simulink model "IDVDSGRA_StatObs_Close"  (R2017b)
settings: Solver=ode4  StartTime=0.0  StopTime=tsim  FixedStep=baseRate  RelTol=1e-3  EnableMultiTasking=on
values from neighbouring files (symbols this model uses):
  baseRate = 0.05    [Run_Initializer.m]
  dockDist = 0.5    [Run_Initializer.m]
  drop_states_BLACK = [ 1.19; 1.45; -0.06737]    [Run_Initializer.m]
  drop_states_RED = [ 2.114; 1.46; -3.113]    [Run_Initializer.m]
  F_thrusters_BLACK = 0.25.*ones(8,1)    [Run_Initializer.m]
  F_thrusters_RED = 0.25.*ones(8,1)    [Run_Initializer.m]
  final_states_BLACK = [1; 0.5; (0/180*pi)]    [Run_Initializer.m]
  fixed_att = init_states_RED(3)    [Run_Initializer.m]
  guess = [8.968203153403679e+02,-2.543974115068790e+03,0.235869606391541,0.474952865321742,0.474987768379695,0.520000000000000,0.485664087948638,0,0,.1,.1,.1,.1,.1,.1,.1,.1,.1,.1,.1,.1,.1,.1,.1,.1,.1,.2]    [Run_Initializer.m]
  home_states_BLACK = [ xLength/2; yLength/2; 0]    [Run_Initializer.m]
  home_states_RED = [ xLength/2+0.4; yLength/2; pi]    [Run_Initializer.m]
  init_states_BLACK = [0.5; 0.5; (0/180*pi)]    [Run_Initializer.m]
  init_states_RED = [ 3; 2; 0]    [Run_Initializer.m]
  Kd_tb = 0.4    [Run_Initializer.m]
  Kd_tr = 0.4    [Run_Initializer.m]
  Kd_xb = 5    [Run_Initializer.m]
  Kd_xr = 5    [Run_Initializer.m]
  Kd_yb = 5    [Run_Initializer.m]
  Kd_yr = 5    [Run_Initializer.m]
  Kp_tb = 0.1    [Run_Initializer.m]
  Kp_tr = 0.1    [Run_Initializer.m]
  Kp_xb = 2    [Run_Initializer.m]
  Kp_xr = 2    [Run_Initializer.m]
  Kp_yb = 2    [Run_Initializer.m]
  Kp_yr = 2    [Run_Initializer.m]
  max_force = F_thrusters_RED(1)*2 * 0.95    [Run_Initializer.m]
  max_torque = 0.13*4    (= 0.52)    [Run_Initializer.m]
  moving_BLACK = [(final_states_BLACK(1)-init_states_BLACK(1))/Phase3_SubPhase2_Duration,(final_states_BLACK(2)-init_states_BLACK(2))/Phase3_SubPhase2_Duration,0]    [Run_Initializer.m]
  noise_variance_BLACK = 0    [Run_Initializer.m]
  noise_variance_RED = 0    [Run_Initializer.m]
  Phase0_End = Phase0_Duration    (= 10)    [Run_Initializer.m]
  Phase1_End = Phase0_Duration + Phase1_Duration    (= 15)    [Run_Initializer.m]
  Phase2_End = Phase0_Duration + Phase1_Duration +                                   Phase2_Duration    (= 35)    [Run_Initializer.m]
  Phase3_Duration = 85    [Run_Initializer.m]
  Phase3_End = Phase0_Duration + Phase1_Duration +                                   Phase2_Duration + Phase3_Duration    (= 120)    [Run_Initializer.m]
  Phase3_SubPhase1_End = Phase2_End + Phase3_SubPhase1_Duration    (= 40)    [Run_Initializer.m]
  Phase3_SubPhase2_Duration = 70    [Run_Initializer.m]
  Phase3_SubPhase2_End = Phase2_End + Phase3_SubPhase1_Duration +                                   Phase3_SubPhase2_Duration    (= 110)    [Run_Initializer.m]
  Phase3_SubPhase3_End = Phase2_End + Phase3_SubPhase1_Duration +                                   Phase3_SubPhase2_Duration +                                  Phase3_SubPhase3_Duration    (= 120)    [Run_Initializer.m]
  Phase3_SubPhase4_End = Phase2_End + Phase3_SubPhase1_Duration +                                   Phase3_SubPhase2_Duration +                                  Phase3_SubPhase3_Duration +                                  Phase3_SubPhase4_Duration    [Run_Initializer.m]
  Phase4_End = Phase0_Duration + Phase1_Duration +                                   Phase2_Duration + Phase3_Duration +                                   Phase4_Duration    (= 140)    [Run_Initializer.m]
  Phase5_End = Phase0_Duration + Phase1_Duration +                                   Phase2_Duration + Phase3_Duration +                                   Phase4_Duration + Phase5_Duration    (= 145)    [Run_Initializer.m]
  REDInertia = 0.2709    [Run_Initializer.m]
  REDMass = 16.9478    [Run_Initializer.m]
  serverRate = 0.1    [Run_Initializer.m]
  thruster_dist2CG_BLACK = [83.42;-52.58;55.94;-60.05;54.08;-53.92;77.06;-55.94]    [Run_Initializer.m]
  thruster_dist2CG_RED = [49.92;-78.08;70.46;-63.54;81.08;-50.42;57.44;-75.96]    [Run_Initializer.m]
  tolSGRA = [Er; Eg]    [Run_Initializer.m]
  xLength = 3.51155    [Run_Initializer.m]
  yLength = 2.41935    [Run_Initializer.m]
undefined symbols (not defined in the file or in its folder): DiscIntNeverNeededParam, platformSelection, simMode
libraries: MainLibrary x22, GPIOLibrary x20, raspberrypilib x17, embdlinuxlib x6, dspsigops x5, dspswit3 x2, simulink x1
(part 7 of 8)

== matlab function IDVDSGRA_StatObs_Close/Phase #3: Experiment/Change RED Behavior/Sub-Phase #2 /Embedded MATLAB Function4 ==
  data: fixed_att input; F output; dock input; cha input; tar input; r0 input; tol input; r output; s input; F0 input; Tmax input; timein input
function [F,r]=IDVD3SGRA(fixed_att, dock,cha,tar,r0,tol,s,F0,Tmax,timein)

%% Definitions of variables
% g = performance index = the manoeuvre's energy [1x1]
% gg = gradient of g [8x1]
% h = constraints [5x1]
% hg = gradient of constraints [8x5]
% g and h are irt varied parameters, r
% r = [d1, d2, tauf, e_FX, e_FY, e_TZ, u, e_t, a4-a9, b4-b9, c4-c9] =[1x26]

% P = constraint error
% E = restoration tolerance 
% cha = chaser's position and velocity [x,y,theta, vx, vy, theta_dot]
% tar = target's position and velocity [x,y,theta, vx, vy, theta_dot]
% dock = docking variables [mass, Ix, FXmax, FYmax, FZmax, docking distance]


if s==0 && Tmax-timein > 1

    Er=tol(1);Eg=tol(2);
    if Tmax-timein>2
        RemTime=Tmax-timein;
    else
        RemTime=2;
    end
    

    par=[dock;cha;tar;RemTime;fixed_att];% Collect all variables in one vector
    
    % Initial Setup
    h = findh(r0, par); 
    P = h' * h;
    Q = 1;
    r=r0;
    
    % Check if Restoration Needed
    if P > Er
            [r, P, Q] = restoration(r, par, P, Er);
    end
  
    % Sequential Algorithm
    loop = 0;
    r_best = r;
    Q_best = Q;

    while loop < 4
        loop = loop + 1;
        [r,P,Q] = gradient(r, par, P, Eg, Q);

        if P > Er
            [r, P, Q] = restoration(r, par, P, Er);
        end

        if (Q < Q_best) && (P <= Er)
            Q_best = Q;
            r_best = r;
        end 
    end
       
    [~,~,~,~,~,~,~,~,F] = final(par, r_best);
    %[tau,t,xt,yt,theta,vx,vy,thetadot,u]=mevalf(par,r_best);
else
    F=zeros(3,1);
    F(1)=F0(1);F(2)=F0(2);F(3)=F0(3);r=r0;
end
end
%%%%%%%%%%%%%%%%%%%%%%%%%%%%%%%%%%%%%%%%%%%%%%%%%%%%%%%%%%%%%%%%%%%%%%%%%%%
%%%%%%%%%%%%%%%%%%%%%%%%%%%%%%%%%%%%%%%%%%%%%%%%%%%%%%%%%%%%%%%%%%%%%%%%%%%
function [r, P, Q] = restoration(r, par, P, Er)
%% Restoration Phase
q=0;
while (P>Er) && (q<10)
    q=q+1;          % counter -> don't do more than 10 iterations
    
    hg = findhg(r, par);
    h = findh(r, par);
    alfa = (hg' * hg) \ h;          % Lagrange multiplier except for the scaling factor, k
    s_delta = -hg * alfa;           % displacement

    k = 1;                          % scaling factor
    qa = 1;
    rp = r + k*s_delta;
    h = findh(rp, par);
    Pp = h'*h;

    while (Pp >= P) && (qa <5)      % using bisection method
        qa = qa +1;                 % only do max 4 iterations
        k = k / 2;
        rp = r + k*s_delta;
        h = findh(rp, par);
        Pp = h'*h;
    end
    r=rp;
    P=Pp;
end

gg = findgg(r, par);
hg = findhg(r, par);
lambda = -(hg' * hg) \ (hg' * gg);
G = gg + hg*lambda;
Q = G' * G;
       
end 
function [r,P,Q] = gradient(r, par, P, Eg, Q)
%% Gradient Phase
count = 0; 
while (Q>Eg) && (count <3)
    count = count + 1;          % no more than 3 iterations   
    
    gg = findgg(r, par);
    hg = findhg(r, par);
    lambda = -(hg' * hg) \ (hg' * gg);
    G = gg + (hg * lambda);
    Q = G' * G;
    
    alfa = 0;
    da = 0.02; 
    
    % Need to find when psi = 0 to find the step size alpha(alfa)
    psi1 = (findgg(r-alfa.*G, par) + (findhg(r-alfa.*G, par)*lambda))' * G ;
    psi2 = (findgg(r-(alfa+da)*G, par) + (findhg(r-(alfa+da)*G, par)*lambda))' * G ;
    
    while (sign(psi1)== sign(psi2)) && (alfa<100) 
        da=da+da^1.3;
        alfa=alfa+da;
        psi1=psi2;
        psi2 = (findgg(r-(alfa+da)*G, par) + (findhg(r-(alfa+da)*G, par)*lambda))' * G ;
    end
    
    alfa = (alfa*psi2 -(alfa+da)*psi1)/(psi2-psi1); % Linear interpolation
    if alfa <= 0         % cannot be a negative number; if it is, set to 1
        alfa = 1;
    end
    
    s = r - alfa*G;
    h = findh(s, par);
    P = h'*h;
    
    Ftilde0 = findg(r, par) + lambda' * findh(r, par);
    count2 = 0;
    hp = h;
    while ((findg(s, par)+lambda'*hp) >= Ftilde0 || P > 10) && (count2<5)
        count2 = count2 + 1;
        alfa = alfa/2;
        s = r-alfa*G;
        hp = findh(s, par);
        P = hp'*hp;
    end    
   
    r = s;
    hg = findhg(r, par);
    gg = findgg(r, par);
    lambda = -(hg' * hg) \ (hg' * gg);
    G = gg + (hg * lambda);
    Q = G' * G;
end  
end 
function [TAU,t,xt,yt,theta,vx,vy,om,F] = final(par, r)
% Performs the final calculations to determine the required thruster
% force in each direction

% Separating out the inputs (computational efficiency)
m=par(1);Iz=par(2);FXmax=par(3);FYmax=par(4);FZmax=par(5);dd=par(6); 
cx=par(7);cy=par(8);cz=par(9);cx_2=par(10);cy_2=par(11);cz_2=par(12);
tx=par(13);ty=par(14);tz=par(15);tx_2=par(16);ty_2=par(17);tz_2=par(18);
Tmax=par(19);fixed_att=par(20);

d1 = r(1); d2 = r(2); tauf = r(3); 
x4=r(9); x5=r(10); x6=r(11); x7=r(12); x8=r(13); x9=r(14);
y4=r(15); y5=r(16); y6=r(17); y7=r(18); y8=r(19); y9=r(20);
z4=r(21); z5=r(22); z6=r(23); z7=r(24); z8=r(25); z9=r(26);

% Initializing 
N=100;
deltaTau = tauf/N;
TAU = zeros(1,N+1);
for i= 2:N+1
    TAU(i) = TAU(i-1) + deltaTau;
end

t=zeros(1,N+1);xt=zeros(1,N+1);yt=zeros(1,N+1);theta=zeros(1,N+1);vx=zeros(1,N+1);
vy=zeros(1,N+1);om=zeros(1,N+1);Fix=zeros(1,N+1);Fiy=zeros(1,N+1);Tz=zeros(1,N+1);

% These equations are the exact same as Marco's (comparison sake), will
% update later
for i = 1:N+1
    tau=TAU(i);
    t(i)=d1*tau+d2*tau^2;
%     xt(i)=cx+cx_2*d1*tau+1/2*(-4*cx_2*d1*tauf-6*cx+6*tx+6*tx_2*(d1*tauf+d2*tauf^2)+6*dd*cos(tz+tz_2*(d1*tauf+d2*tauf^2))-2*tauf*(tx_2-tz_2*dd*sin(tz+tz_2*(d1*tauf+d2*tauf^2)))*(d1+2*d2*tauf))/tauf^2*tau^2+1/6*(12*cx+6*cx_2*d1*tauf-12*tx-12*tx_2*(d1*tauf+d2*tauf^2)-12*dd*cos(tz+tz_2*(d1*tauf+d2*tauf^2))+6*tauf*(tx_2-tz_2*dd*sin(tz+tz_2*(d1*tauf+d2*tauf^2)))*(d1+2*d2*tauf))/tauf^3*tau^3;
%     yt(i)=cy+cy_2*d1*tau+1/2*(-4*cy_2*d1*tauf-6*cy+6*ty+6*ty_2*(d1*tauf+d2*tauf^2)+6*dd*sin(tz+tz_2*(d1*tauf+d2*tauf^2))-2*tauf*(ty_2+tz_2*dd*cos(tz+tz_2*(d1*tauf+d2*tauf^2)))*(d1+2*d2*tauf))/tauf^2*tau^2+1/6*(12*cy+6*cy_2*d1*tauf-12*ty-12*ty_2*(d1*tauf+d2*tauf^2)-12*dd*sin(tz+tz_2*(d1*tauf+d2*tauf^2))+6*tauf*(ty_2+tz_2*dd*cos(tz+tz_2*(d1*tauf+d2*tauf^2)))*(d1+2*d2*tauf))/tauf^3*tau^3;
%     theta(i)=cz+cz_2*d1*tau+1/2*(-4*cz_2*d1*tauf-6*cz+6*tz+6*tz_2*(d1*tauf+d2*tauf^2)-2*tauf*tz_2*(d1+2*d2*tauf))/tauf^2*tau^2+1/6*(12*cz+6*cz_2*d1*tauf-12*tz-12*tz_2*(d1*tauf+d2*tauf^2)+6*tauf*tz_2*(d1+2*d2*tauf))/tauf^3*tau^3;
%     vx(i)=(cx_2*d1+(-4*cx_2*d1*tauf-6*cx+6*tx+6*tx_2*(d1*tauf+d2*tauf^2)+6*dd*cos(tz+tz_2*(d1*tauf+d2*tauf^2))-2*tauf*(tx_2-tz_2*dd*sin(tz+tz_2*(d1*tauf+d2*tauf^2)))*(d1+2*d2*tauf))/tauf^2*tau+1/2*(12*cx+6*cx_2*d1*tauf-12*tx-12*tx_2*(d1*tauf+d2*tauf^2)-12*dd*cos(tz+tz_2*(d1*tauf+d2*tauf^2))+6*tauf*(tx_2-tz_2*dd*sin(tz+tz_2*(d1*tauf+d2*tauf^2)))*(d1+2*d2*tauf))/tauf^3*tau^2)/(d1+2*d2*tau);
%     vy(i)=(cy_2*d1+(-4*cy_2*d1*tauf-6*cy+6*ty+6*ty_2*(d1*tauf+d2*tauf^2)+6*dd*sin(tz+tz_2*(d1*tauf+d2*tauf^2))-2*tauf*(ty_2+tz_2*dd*cos(tz+tz_2*(d1*tauf+d2*tauf^2)))*(d1+2*d2*tauf))/tauf^2*tau+1/2*(12*cy+6*cy_2*d1*tauf-12*ty-12*ty_2*(d1*tauf+d2*tauf^2)-12*dd*sin(tz+tz_2*(d1*tauf+d2*tauf^2))+6*tauf*(ty_2+tz_2*dd*cos(tz+tz_2*(d1*tauf+d2*tauf^2)))*(d1+2*d2*tauf))/tauf^3*tau^2)/(d1+2*d2*tau);
%     om(i)=(cz_2*d1+(-4*cz_2*d1*tauf-6*cz+6*tz+6*tz_2*(d1*tauf+d2*tauf^2)-2*tauf*tz_2*(d1+2*d2*tauf))/tauf^2*tau+1/2*(12*cz+6*cz_2*d1*tauf-12*tz-12*tz_2*(d1*tauf+d2*tauf^2)+6*tauf*tz_2*(d1+2*d2*tauf))/tauf^3*tau^2)/(d1+2*d2*tau);
%     Fix(i)=-2*m*(2*cx_2*d1^2*tauf^2-2*tx_2*tauf^2*d1^2-6*tau^2*cx*d2+6*tau^2*tx*d2+3*tauf*cx*d1-3*tauf*tx*d1-6*tau*cx*d1+6*tau*tx*d1-tauf^2*tz_2*dd*sin(tz+tz_2*d1*tauf+tz_2*d2*tauf^2)*d1^2+6*tauf^2*tz_2*dd*sin(tz+tz_2*d1*tauf+tz_2*d2*tauf^2)*d1*d2*tau-3*tau^2*cx_2*d1*tauf*d2+3*tau^2*tx_2*tauf*d1*d2+3*tau*tauf*tz_2*dd*sin(tz+tz_2*d1*tauf+tz_2*d2*tauf^2)*d1^2+3*tau^2*tauf*tz_2*dd*sin(tz+tz_2*d1*tauf+tz_2*d2*tauf^2)*d1*d2+6*tau^2*tz_2*dd*sin(tz+tz_2*d1*tauf+tz_2*d2*tauf^2)*d2^2*tauf^2-2*tz_2*dd*sin(tz+tz_2*d1*tauf+tz_2*d2*tauf^2)*d2*tauf^3*d1-3*tau*cx_2*d1^2*tauf+3*tau*tx_2*tauf*d1^2+6*tau^2*dd*cos(tz+tz_2*d1*tauf+tz_2*d2*tauf^2)*d2-tx_2*tauf^3*d2*d1-3*tauf*dd*cos(tz+tz_2*d1*tauf+tz_2*d2*tauf^2)*d1+6*tau*dd*cos(tz+tz_2*d1*tauf+tz_2*d2*tauf^2)*d1+d2*cx_2*d1*tauf^3)/tauf^3/(d1+2*d2*tau)^3;
%     Fiy(i)=2*m*(-2*cy_2*d1^2*tauf^2+2*ty_2*tauf^2*d1^2+6*tau^2*cy*d2-6*tau^2*ty*d2-3*tauf*cy*d1+3*tauf*ty*d1+6*tau*cy*d1-6*tau*ty*d1+3*tau*cy_2*d1^2*tauf-3*tau*ty_2*tauf*d1^2-6*tau^2*dd*sin(tz+tz_2*d1*tauf+tz_2*d2*tauf^2)*d2+ty_2*tauf^3*d2*d1+3*tauf*dd*sin(tz+tz_2*d1*tauf+tz_2*d2*tauf^2)*d1-6*tau*dd*sin(tz+tz_2*d1*tauf+tz_2*d2*tauf^2)*d1-d2*cy_2*d1*tauf^3-tauf^2*tz_2*dd*cos(tz+tz_2*d1*tauf+tz_2*d2*tauf^2)*d1^2+6*tauf^2*tz_2*dd*cos(tz+tz_2*d1*tauf+tz_2*d2*tauf^2)*d1*d2*tau+3*tau^2*cy_2*d1*tauf*d2-3*tau^2*ty_2*tauf*d1*d2+3*tau*tauf*tz_2*dd*cos(tz+tz_2*d1*tauf+tz_2*d2*tauf^2)*d1^2+3*tau^2*tauf*tz_2*dd*cos(tz+tz_2*d1*tauf+tz_2*d2*tauf^2)*d1*d2+6*tau^2*tz_2*dd*cos(tz+tz_2*d1*tauf+tz_2*d2*tauf^2)*d2^2*tauf^2-2*tz_2*dd*cos(tz+tz_2*d1*tauf+tz_2*d2*tauf^2)*d2*tauf^3*d1)/tauf^3/(d1+2*d2*tau)^3;
%     Tz(i)=-2*Iz*(-3*tau*cz_2*d1^2*tauf+3*tau*tz_2*d1^2*tauf-tz_2*d2*tauf^3*d1+d2*cz_2*d1*tauf^3+3*tau^2*tz_2*d1*tauf*d2-3*tau^2*cz_2*d1*tauf*d2+2*cz_2*d1^2*tauf^2-2*tz_2*d1^2*tauf^2-6*tau^2*cz*d2+6*tau^2*tz*d2+3*tauf*cz*d1-3*tauf*tz*d1-6*tau*cz*d1+6*tau*tz*d1)/tauf^3/(d1+2*d2*tau)^3;
     % theta(i)= cz + ((d2*tau^2 + d1*tau)^3*(2*cz - 2*tz + 2*tauf^4*z4 + 2*tauf^5*z5 + 2*tauf^6*z6 + 2*tauf^7*z7 + 2*tauf^8*z8 + 2*tauf^9*z9 + cz_2*d1*tauf - d1*tauf*tz_2))/tauf^3 - ((d2*tau^2 + d1*tau)^2*(3*cz - 3*tz + 3*tauf^4*z4 + 3*tauf^5*z5 + 3*tauf^6*z6 + 3*tauf^7*z7 + 3*tauf^8*z8 + 3*tauf^9*z9 - d2*tauf^2*tz_2 + 2*cz_2*d1*tauf - 2*d1*tauf*tz_2))/tauf^2 + cz_2*d1*(d2*tau^2 + d1*tau);
     % Fix(i)= -m*(((30*cx - 30*tx + 30*tauf^4*x4 + 30*tauf^5*x5 + 30*tauf^6*x6 + 30*tauf^7*x7 + 30*tauf^8*x8 + 30*tauf^9*x9 - 30*dd*cos(tz + tz_2*(d2*tauf^2 + d1*tauf)) + 11*d2*tauf^2*tx_2 + 20*cx_2*d1*tauf + d1*tauf*tx_2 - 10*d1*dd*tauf*tz_2*sin(tz + tz_2*(d2*tauf^2 + d1*tauf)) - 20*d2*dd*tauf^2*tz_2*sin(tz + tz_2*(d2*tauf^2 + d1*tauf)))/(5*tauf^2) - (6*tau*(10*cx - 10*tx + 10*tauf^4*x4 + 10*tauf^5*x5 + 10*tauf^6*x6 + 10*tauf^7*x7 + 10*tauf^8*x8 + 10*tauf^9*x9 - 10*dd*cos(tz + tz_2*(d2*tauf^2 + d1*tauf)) + 7*d2*tauf^2*tx_2 + 5*cx_2*d1*tauf + 2*d1*tauf*tx_2 - 5*d1*dd*tauf*tz_2*sin(tz + tz_2*(d2*tauf^2 + d1*tauf)) - 10*d2*dd*tauf^2*tz_2*sin(tz + tz_2*(d2*tauf^2 + d1*tauf))))/(5*tauf^3))/(d1 + 2*d2*tau)^2 + (2*d2*(cx_2*d1 - (tau*(30*cx - 30*tx + 30*tauf^4*x4 + 30*tauf^5*x5 + 30*tauf^6*x6 + 30*tauf^7*x7 + 30*tauf^8*x8 + 30*tauf^9*x9 - 30*dd*cos(tz + tz_2*(d2*tauf^2 + d1*tauf)) + 11*d2*tauf^2*tx_2 + 20*cx_2*d1*tauf + d1*tauf*tx_2 - 10*d1*dd*tauf*tz_2*sin(tz + tz_2*(d2*tauf^2 + d1*tauf)) - 20*d2*dd*tauf^2*tz_2*sin(tz + tz_2*(d2*tauf^2 + d1*tauf))))/(5*tauf^2) + (3*tau^2*(10*cx - 10*tx + 10*tauf^4*x4 + 10*tauf^5*x5 + 10*tauf^6*x6 + 10*tauf^7*x7 + 10*tauf^8*x8 + 10*tauf^9*x9 - 10*dd*cos(tz + tz_2*(d2*tauf^2 + d1*tauf)) + 7*d2*tauf^2*tx_2 + 5*cx_2*d1*tauf + 2*d1*tauf*tx_2 - 5*d1*dd*tauf*tz_2*sin(tz + tz_2*(d2*tauf^2 + d1*tauf)) - 10*d2*dd*tauf^2*tz_2*sin(tz + tz_2*(d2*tauf^2 + d1*tauf))))/(5*tauf^3)))/(d1 + 2*d2*tau)^3);
     % Fiy(i)= -m*(((30*cy - 30*ty - 30*dd*sin(tz + tz_2*(d2*tauf^2 + d1*tauf)) + 30*tauf^4*y4 + 30*tauf^5*y5 + 30*tauf^6*y6 + 30*tauf^7*y7 + 30*tauf^8*y8 + 30*tauf^9*y9 + 11*d2*tauf^2*ty_2 + 20*cy_2*d1*tauf + d1*tauf*ty_2 + 10*d1*dd*tauf*tz_2*sin(tz + tz_2*(d2*tauf^2 + d1*tauf)) + 20*d2*dd*tauf^2*tz_2*sin(tz + tz_2*(d2*tauf^2 + d1*tauf)))/(5*tauf^2) - (6*tau*(10*cy - 10*ty - 10*dd*sin(tz + tz_2*(d2*tauf^2 + d1*tauf)) + 10*tauf^4*y4 + 10*tauf^5*y5 + 10*tauf^6*y6 + 10*tauf^7*y7 + 10*tauf^8*y8 + 10*tauf^9*y9 + 7*d2*tauf^2*ty_2 + 5*cy_2*d1*tauf + 2*d1*tauf*ty_2 + 5*d1*dd*tauf*tz_2*sin(tz + tz_2*(d2*tauf^2 + d1*tauf)) + 10*d2*dd*tauf^2*tz_2*sin(tz + tz_2*(d2*tauf^2 + d1*tauf))))/(5*tauf^3))/(d1 + 2*d2*tau)^2 + (2*d2*(cy_2*d1 - (tau*(30*cy - 30*ty - 30*dd*sin(tz + tz_2*(d2*tauf^2 + d1*tauf)) + 30*tauf^4*y4 + 30*tauf^5*y5 + 30*tauf^6*y6 + 30*tauf^7*y7 + 30*tauf^8*y8 + 30*tauf^9*y9 + 11*d2*tauf^2*ty_2 + 20*cy_2*d1*tauf + d1*tauf*ty_2 + 10*d1*dd*tauf*tz_2*sin(tz + tz_2*(d2*tauf^2 + d1*tauf)) + 20*d2*dd*tauf^2*tz_2*sin(tz + tz_2*(d2*tauf^2 + d1*tauf))))/(5*tauf^2) + (3*tau^2*(10*cy - 10*ty - 10*dd*sin(tz + tz_2*(d2*tauf^2 + d1*tauf)) + 10*tauf^4*y4 + 10*tauf^5*y5 + 10*tauf^6*y6 + 10*tauf^7*y7 + 10*tauf^8*y8 + 10*tauf^9*y9 + 7*d2*tauf^2*ty_2 + 5*cy_2*d1*tauf + 2*d1*tauf*ty_2 + 5*d1*dd*tauf*tz_2*sin(tz + tz_2*(d2*tauf^2 + d1*tauf)) + 10*d2*dd*tauf^2*tz_2*sin(tz + tz_2*(d2*tauf^2 + d1*tauf))))/(5*tauf^3)))/(d1 + 2*d2*tau)^3);
     % Tz(i)= -Iz*(((2*(3*cz - 3*tz + 3*tauf^4*z4 + 3*tauf^5*z5 + 3*tauf^6*z6 + 3*tauf^7*z7 + 3*tauf^8*z8 + 3*tauf^9*z9 - d2*tauf^2*tz_2 + 2*cz_2*d1*tauf - 2*d1*tauf*tz_2))/tauf^2 - (6*tau*(2*cz - 2*tz + 2*tauf^4*z4 + 2*tauf^5*z5 + 2*tauf^6*z6 + 2*tauf^7*z7 + 2*tauf^8*z8 + 2*tauf^9*z9 + cz_2*d1*tauf - d1*tauf*tz_2))/tauf^3)/(d1 + 2*d2*tau)^2 + (2*d2*(cz_2*d1 - (2*tau*(3*cz - 3*tz + 3*tauf^4*z4 + 3*tauf^5*z5 + 3*tauf^6*z6 + 3*tauf^7*z7 + 3*tauf^8*z8 + 3*tauf^9*z9 - d2*tauf^2*tz_2 + 2*cz_2*d1*tauf - 2*d1*tauf*tz_2))/tauf^2 + (3*tau^2*(2*cz - 2*tz + 2*tauf^4*z4 + 2*tauf^5*z5 + 2*tauf^6*z6 + 2*tauf^7*z7 + 2*tauf^8*z8 + 2*tauf^9*z9 + cz_2*d1*tauf - d1*tauf*tz_2))/tauf^3))/(d1 + 2*d2*tau)^3);
theta(i)= cz + ((d2*tau^2 + d1*tau)^3*(2*cz - 2*tz + 2*tauf^4*z4 + 2*tauf^5*z5 + 2*tauf^6*z6 + 2*tauf^7*z7 + 2*tauf^8*z8 + 2*tauf^9*z9 + cz_2*d1*tauf - d1*tauf*tz_2))/tauf^3 - ((d2*tau^2 + d1*tau)^2*(3*cz - 3*tz + 3*tauf^4*z4 + 3*tauf^5*z5 + 3*tauf^6*z6 + 3*tauf^7*z7 + 3*tauf^8*z8 + 3*tauf^9*z9 - d2*tauf^2*tz_2 + 2*cz_2*d1*tauf - 2*d1*tauf*tz_2))/tauf^2 + cz_2*d1*(d2*tau^2 + d1*tau);
      Fix(i)= -m*(((2*(3*cx - 3*tx + 3*tauf^4*x4 + 3*tauf^5*x5 + 3*tauf^6*x6 + 3*tauf^7*x7 + 3*tauf^8*x8 + 3*tauf^9*x9 - 3*dd*cos(tz + tz_2*(d2*tauf^2 + d1*tauf)) - d2*tauf^2*tx_2 + 2*cx_2*d1*tauf - 2*d1*tauf*tx_2 - d1*dd*tauf*tz_2*sin(tz + tz_2*(d2*tauf^2 + d1*tauf)) - 2*d2*dd*tauf^2*tz_2*sin(tz + tz_2*(d2*tauf^2 + d1*tauf))))/tauf^2 - (6*tau*(2*cx - 2*tx + 2*tauf^4*x4 + 2*tauf^5*x5 + 2*tauf^6*x6 + 2*tauf^7*x7 + 2*tauf^8*x8 + 2*tauf^9*x9 - 2*dd*cos(tz + tz_2*(d2*tauf^2 + d1*tauf)) + cx_2*d1*tauf - d1*tauf*tx_2 - d1*dd*tauf*tz_2*sin(tz + tz_2*(d2*tauf^2 + d1*tauf)) - 2*d2*dd*tauf^2*tz_2*sin(tz + tz_2*(d2*tauf^2 + d1*tauf))))/tauf^3)/(d1 + 2*d2*tau)^2 + (2*d2*(cx_2*d1 - (2*tau*(3*cx - 3*tx + 3*tauf^4*x4 + 3*tauf^5*x5 + 3*tauf^6*x6 + 3*tauf^7*x7 + 3*tauf^8*x8 + 3*tauf^9*x9 - 3*dd*cos(tz + tz_2*(d2*tauf^2 + d1*tauf)) - d2*tauf^2*tx_2 + 2*cx_2*d1*tauf - 2*d1*tauf*tx_2 - d1*dd*tauf*tz_2*sin(tz + tz_2*(d2*tauf^2 + d1*tauf)) - 2*d2*dd*tauf^2*tz_2*sin(tz + tz_2*(d2*tauf^2 + d1*tauf))))/tauf^2 + (3*tau^2*(2*cx - 2*tx + 2*tauf^4*x4 + 2*tauf^5*x5 + 2*tauf^6*x6 + 2*tauf^7*x7 + 2*tauf^8*x8 + 2*tauf^9*x9 - 2*dd*cos(tz + tz_2*(d2*tauf^2 + d1*tauf)) + cx_2*d1*tauf - d1*tauf*tx_2 - d1*dd*tauf*tz_2*sin(tz + tz_2*(d2*tauf^2 + d1*tauf)) - 2*d2*dd*tauf^2*tz_2*sin(tz + tz_2*(d2*tauf^2 + d1*tauf))))/tauf^3))/(d1 + 2*d2*tau)^3);
      Fiy(i)= -m*(((2*(3*cy - 3*ty - 3*dd*sin(tz + tz_2*(d2*tauf^2 + d1*tauf)) + 3*tauf^4*y4 + 3*tauf^5*y5 + 3*tauf^6*y6 + 3*tauf^7*y7 + 3*tauf^8*y8 + 3*tauf^9*y9 - d2*tauf^2*ty_2 + 2*cy_2*d1*tauf - 2*d1*tauf*ty_2 + d1*dd*tauf*tz_2*sin(tz + tz_2*(d2*tauf^2 + d1*tauf)) + 2*d2*dd*tauf^2*tz_2*sin(tz + tz_2*(d2*tauf^2 + d1*tauf))))/tauf^2 - (6*tau*(2*cy - 2*ty - 2*dd*sin(tz + tz_2*(d2*tauf^2 + d1*tauf)) + 2*tauf^4*y4 + 2*tauf^5*y5 + 2*tauf^6*y6 + 2*tauf^7*y7 + 2*tauf^8*y8 + 2*tauf^9*y9 + cy_2*d1*tauf - d1*tauf*ty_2 + d1*dd*tauf*tz_2*sin(tz + tz_2*(d2*tauf^2 + d1*tauf)) + 2*d2*dd*tauf^2*tz_2*sin(tz + tz_2*(d2*tauf^2 + d1*tauf))))/tauf^3)/(d1 + 2*d2*tau)^2 + (2*d2*(cy_2*d1 - (2*tau*(3*cy - 3*ty - 3*dd*sin(tz + tz_2*(d2*tauf^2 + d1*tauf)) + 3*tauf^4*y4 + 3*tauf^5*y5 + 3*tauf^6*y6 + 3*tauf^7*y7 + 3*tauf^8*y8 + 3*tauf^9*y9 - d2*tauf^2*ty_2 + 2*cy_2*d1*tauf - 2*d1*tauf*ty_2 + d1*dd*tauf*tz_2*sin(tz + tz_2*(d2*tauf^2 + d1*tauf)) + 2*d2*dd*tauf^2*tz_2*sin(tz + tz_2*(d2*tauf^2 + d1*tauf))))/tauf^2 + (3*tau^2*(2*cy - 2*ty - 2*dd*sin(tz + tz_2*(d2*tauf^2 + d1*tauf)) + 2*tauf^4*y4 + 2*tauf^5*y5 + 2*tauf^6*y6 + 2*tauf^7*y7 + 2*tauf^8*y8 + 2*tauf^9*y9 + cy_2*d1*tauf - d1*tauf*ty_2 + d1*dd*tauf*tz_2*sin(tz + tz_2*(d2*tauf^2 + d1*tauf)) + 2*d2*dd*tauf^2*tz_2*sin(tz + tz_2*(d2*tauf^2 + d1*tauf))))/tauf^3))/(d1 + 2*d2*tau)^3);
      Tz(i)= -Iz*(((2*(3*cz - 3*tz + 3*tauf^4*z4 + 3*tauf^5*z5 + 3*tauf^6*z6 + 3*tauf^7*z7 + 3*tauf^8*z8 + 3*tauf^9*z9 - d2*tauf^2*tz_2 + 2*cz_2*d1*tauf - 2*d1*tauf*tz_2))/tauf^2 - (6*tau*(2*cz - 2*tz + 2*tauf^4*z4 + 2*tauf^5*z5 + 2*tauf^6*z6 + 2*tauf^7*z7 + 2*tauf^8*z8 + 2*tauf^9*z9 + cz_2*d1*tauf - d1*tauf*tz_2))/tauf^3)/(d1 + 2*d2*tau)^2 + (2*d2*(cz_2*d1 - (2*tau*(3*cz - 3*tz + 3*tauf^4*z4 + 3*tauf^5*z5 + 3*tauf^6*z6 + 3*tauf^7*z7 + 3*tauf^8*z8 + 3*tauf^9*z9 - d2*tauf^2*tz_2 + 2*cz_2*d1*tauf - 2*d1*tauf*tz_2))/tauf^2 + (3*tau^2*(2*cz - 2*tz + 2*tauf^4*z4 + 2*tauf^5*z5 + 2*tauf^6*z6 + 2*tauf^7*z7 + 2*tauf^8*z8 + 2*tauf^9*z9 + cz_2*d1*tauf - d1*tauf*tz_2))/tauf^3))/(d1 + 2*d2*tau)^3);
    
end

Fx = Fix.*cos(theta) + Fiy.*sin(theta);
Fy = -Fix.*sin(theta) + Fiy.*cos(theta);

if Fx(1)>FXmax
    Fx(1)=FXmax;
elseif  Fx(1)<-FXmax
    Fx(1)=-FXmax;
end

if Fy(1)>FYmax
    Fy(1)=FYmax;
elseif  Fy(1)<-FYmax
    Fy(1)=-FYmax;
end

if Tz(1)>FZmax
    Tz(1)=FZmax;
elseif  Tz(1)<-FZmax
    Tz(1)=-FZmax;
end

F=[Fx(1) Fy(1) Tz(1)]';

end
%%%%%%%%%%%%%%%%%%%%%%%%%%%%%%%%%%%%%%%%%%%%%%%%%%%%%%%%%%%%%%%%%%%%%%%%%%%
function g = findg(r, par)
% This function calculates the performance index 
%
% Inputs:
%   - r = varied parameters = [d1, d2, tauf, e_FX, e_FY, e_TZ, u, e_t]
%   - cha = conditions of chaser 'initial' [x,y,z,xv,yv,zv]
%   - tar = conditions of target 'final' [X,Y,Z,XV,YV,ZV]
%   - dock = docking variables [mass, mom_inertia, Fmax, Torque_max, dock_distance,
%            time_remaining]
% Outputs:
%   - g = performace index [1x1]
% Comment: 

% Separating out the inputs (computational efficiency)
m=par(1);Iz=par(2);FXmax=par(3);FYmax=par(4);FZmax=par(5);dd=par(6); 
cx=par(7);cy=par(8);cz=par(9);cx_2=par(10);cy_2=par(11);cz_2=par(12);
tx=par(13);ty=par(14);tz=par(15);tx_2=par(16);ty_2=par(17);tz_2=par(18);
Tmax=par(19);fixed_att=par(20);

d1 = r(1); d2 = r(2); tauf = r(3); e_FX = r(4);
e_FY = r(5); e_TZ = r(6); u = r(7); e_t = r(8);
x4=r(9); x5=r(10); x6=r(11); x7=r(12); x8=r(13); x9=r(14);
y4=r(15); y5=r(16); y6=r(17); y7=r(18); y8=r(19); y9=r(20);
z4=r(21); z5=r(22); z6=r(23); z7=r(24); z8=r(25); z9=r(26);


% Determining the performance index
n=20;
TAU=(0:1/n:1)*tauf;
fx=zeros(1,length(TAU)); fy=zeros(1,length(TAU)); fz=zeros(1,length(TAU)); E=zeros(1,length(TAU));
    
for i=1:length(TAU)
    tau=TAU(i);
    fx(i)= -m*(((30*cx - 30*tx + 30*tauf^4*x4 + 30*tauf^5*x5 + 30*tauf^6*x6 + 30*tauf^7*x7 + 30*tauf^8*x8 + 30*tauf^9*x9 - 30*dd*cos(tz + tz_2*(d2*tauf^2 + d1*tauf)) + 11*d2*tauf^2*tx_2 + 20*cx_2*d1*tauf + d1*tauf*tx_2 - 10*d1*dd*tauf*tz_2*sin(tz + tz_2*(d2*tauf^2 + d1*tauf)) - 20*d2*dd*tauf^2*tz_2*sin(tz + tz_2*(d2*tauf^2 + d1*tauf)))/(5*tauf^2) - (6*tau*(10*cx - 10*tx + 10*tauf^4*x4 + 10*tauf^5*x5 + 10*tauf^6*x6 + 10*tauf^7*x7 + 10*tauf^8*x8 + 10*tauf^9*x9 - 10*dd*cos(tz + tz_2*(d2*tauf^2 + d1*tauf)) + 7*d2*tauf^2*tx_2 + 5*cx_2*d1*tauf + 2*d1*tauf*tx_2 - 5*d1*dd*tauf*tz_2*sin(tz + tz_2*(d2*tauf^2 + d1*tauf)) - 10*d2*dd*tauf^2*tz_2*sin(tz + tz_2*(d2*tauf^2 + d1*tauf))))/(5*tauf^3))/(d1 + 2*d2*tau)^2 + (2*d2*(cx_2*d1 - (tau*(30*cx - 30*tx + 30*tauf^4*x4 + 30*tauf^5*x5 + 30*tauf^6*x6 + 30*tauf^7*x7 + 30*tauf^8*x8 + 30*tauf^9*x9 - 30*dd*cos(tz + tz_2*(d2*tauf^2 + d1*tauf)) + 11*d2*tauf^2*tx_2 + 20*cx_2*d1*tauf + d1*tauf*tx_2 - 10*d1*dd*tauf*tz_2*sin(tz + tz_2*(d2*tauf^2 + d1*tauf)) - 20*d2*dd*tauf^2*tz_2*sin(tz + tz_2*(d2*tauf^2 + d1*tauf))))/(5*tauf^2) + (3*tau^2*(10*cx - 10*tx + 10*tauf^4*x4 + 10*tauf^5*x5 + 10*tauf^6*x6 + 10*tauf^7*x7 + 10*tauf^8*x8 + 10*tauf^9*x9 - 10*dd*cos(tz + tz_2*(d2*tauf^2 + d1*tauf)) + 7*d2*tauf^2*tx_2 + 5*cx_2*d1*tauf + 2*d1*tauf*tx_2 - 5*d1*dd*tauf*tz_2*sin(tz + tz_2*(d2*tauf^2 + d1*tauf)) - 10*d2*dd*tauf^2*tz_2*sin(tz + tz_2*(d2*tauf^2 + d1*tauf))))/(5*tauf^3)))/(d1 + 2*d2*tau)^3);
    fy(i)= -m*(((30*cy - 30*ty - 30*dd*sin(tz + tz_2*(d2*tauf^2 + d1*tauf)) + 30*tauf^4*y4 + 30*tauf^5*y5 + 30*tauf^6*y6 + 30*tauf^7*y7 + 30*tauf^8*y8 + 30*tauf^9*y9 + 11*d2*tauf^2*ty_2 + 20*cy_2*d1*tauf + d1*tauf*ty_2 + 10*d1*dd*tauf*tz_2*sin(tz + tz_2*(d2*tauf^2 + d1*tauf)) + 20*d2*dd*tauf^2*tz_2*sin(tz + tz_2*(d2*tauf^2 + d1*tauf)))/(5*tauf^2) - (6*tau*(10*cy - 10*ty - 10*dd*sin(tz + tz_2*(d2*tauf^2 + d1*tauf)) + 10*tauf^4*y4 + 10*tauf^5*y5 + 10*tauf^6*y6 + 10*tauf^7*y7 + 10*tauf^8*y8 + 10*tauf^9*y9 + 7*d2*tauf^2*ty_2 + 5*cy_2*d1*tauf + 2*d1*tauf*ty_2 + 5*d1*dd*tauf*tz_2*sin(tz + tz_2*(d2*tauf^2 + d1*tauf)) + 10*d2*dd*tauf^2*tz_2*sin(tz + tz_2*(d2*tauf^2 + d1*tauf))))/(5*tauf^3))/(d1 + 2*d2*tau)^2 + (2*d2*(cy_2*d1 - (tau*(30*cy - 30*ty - 30*dd*sin(tz + tz_2*(d2*tauf^2 + d1*tauf)) + 30*tauf^4*y4 + 30*tauf^5*y5 + 30*tauf^6*y6 + 30*tauf^7*y7 + 30*tauf^8*y8 + 30*tauf^9*y9 + 11*d2*tauf^2*ty_2 + 20*cy_2*d1*tauf + d1*tauf*ty_2 + 10*d1*dd*tauf*tz_2*sin(tz + tz_2*(d2*tauf^2 + d1*tauf)) + 20*d2*dd*tauf^2*tz_2*sin(tz + tz_2*(d2*tauf^2 + d1*tauf))))/(5*tauf^2) + (3*tau^2*(10*cy - 10*ty - 10*dd*sin(tz + tz_2*(d2*tauf^2 + d1*tauf)) + 10*tauf^4*y4 + 10*tauf^5*y5 + 10*tauf^6*y6 + 10*tauf^7*y7 + 10*tauf^8*y8 + 10*tauf^9*y9 + 7*d2*tauf^2*ty_2 + 5*cy_2*d1*tauf + 2*d1*tauf*ty_2 + 5*d1*dd*tauf*tz_2*sin(tz + tz_2*(d2*tauf^2 + d1*tauf)) + 10*d2*dd*tauf^2*tz_2*sin(tz + tz_2*(d2*tauf^2 + d1*tauf))))/(5*tauf^3)))/(d1 + 2*d2*tau)^3);
    fz(i)= -Iz*(((2*(3*cz - 3*tz + 3*tauf^4*z4 + 3*tauf^5*z5 + 3*tauf^6*z6 + 3*tauf^7*z7 + 3*tauf^8*z8 + 3*tauf^9*z9 - d2*tauf^2*tz_2 + 2*cz_2*d1*tauf - 2*d1*tauf*tz_2))/tauf^2 - (6*tau*(2*cz - 2*tz + 2*tauf^4*z4 + 2*tauf^5*z5 + 2*tauf^6*z6 + 2*tauf^7*z7 + 2*tauf^8*z8 + 2*tauf^9*z9 + cz_2*d1*tauf - d1*tauf*tz_2))/tauf^3)/(d1 + 2*d2*tau)^2 + (2*d2*(cz_2*d1 - (2*tau*(3*cz - 3*tz + 3*tauf^4*z4 + 3*tauf^5*z5 + 3*tauf^6*z6 + 3*tauf^7*z7 + 3*tauf^8*z8 + 3*tauf^9*z9 - d2*tauf^2*tz_2 + 2*cz_2*d1*tauf - 2*d1*tauf*tz_2))/tauf^2 + (3*tau^2*(2*cz - 2*tz + 2*tauf^4*z4 + 2*tauf^5*z5 + 2*tauf^6*z6 + 2*tauf^7*z7 + 2*tauf^8*z8 + 2*tauf^9*z9 + cz_2*d1*tauf - d1*tauf*tz_2))/tauf^3))/(d1 + 2*d2*tau)^3);
    E(i)=(fx(i)^2+fy(i)^2+fz(i)^2);
end 

g=trapz(TAU,E.*(d1+2*d2*TAU));

end 
function gg = findgg(r,par)

% Separating out the inputs (computational efficiency)
m=par(1);Iz=par(2);FXmax=par(3);FYmax=par(4);FZmax=par(5);dd=par(6); 
cx=par(7);cy=par(8);cz=par(9);cx_2=par(10);cy_2=par(11);cz_2=par(12);
tx=par(13);ty=par(14);tz=par(15);tx_2=par(16);ty_2=par(17);tz_2=par(18);
Tmax=par(19);fixed_att=par(20);

%%
r = r';
r0 = r;
n=20;
D=abs(r/1000)+0.0001;
dg=zeros(1,length(r));
for j=1:length(r)
    rp=r0; rn=r0;
    rp(j)=rp(j)+D(j);rn(j)=rn(j)-D(j);
    rpn=[rp;rn]; 
    Ep=zeros(1,n+1);En=zeros(1,n+1);
    TAU=(0:1/n:1)*r(3);        
    for s=1:2    % run through the loop twice, once for rp and once for rn
        r=rpn(s,:);
        d1 = r(1); d2 = r(2); tauf = r(3); e_FX = r(4);
        e_FY = r(5); e_TZ = r(6); u = r(7); e_t = r(8);
        x4=r(9); x5=r(10); x6=r(11); x7=r(12); x8=r(13); x9=r(14);
        y4=r(15); y5=r(16); y6=r(17); y7=r(18); y8=r(19); y9=r(20);
        z4=r(21); z5=r(22); z6=r(23); z7=r(24); z8=r(25); z9=r(26);
        
        TAU=(0:1/n:1)*tauf;
        fx=zeros(1,length(TAU)); fy=zeros(1,length(TAU)); fz=zeros(1,length(TAU));
        for i=1:length(TAU)
            tau=TAU(i);
            fx(i)= -m*(((30*cx - 30*tx + 30*tauf^4*x4 + 30*tauf^5*x5 + 30*tauf^6*x6 + 30*tauf^7*x7 + 30*tauf^8*x8 + 30*tauf^9*x9 - 30*dd*cos(tz + tz_2*(d2*tauf^2 + d1*tauf)) + 11*d2*tauf^2*tx_2 + 20*cx_2*d1*tauf + d1*tauf*tx_2 - 10*d1*dd*tauf*tz_2*sin(tz + tz_2*(d2*tauf^2 + d1*tauf)) - 20*d2*dd*tauf^2*tz_2*sin(tz + tz_2*(d2*tauf^2 + d1*tauf)))/(5*tauf^2) - (6*tau*(10*cx - 10*tx + 10*tauf^4*x4 + 10*tauf^5*x5 + 10*tauf^6*x6 + 10*tauf^7*x7 + 10*tauf^8*x8 + 10*tauf^9*x9 - 10*dd*cos(tz + tz_2*(d2*tauf^2 + d1*tauf)) + 7*d2*tauf^2*tx_2 + 5*cx_2*d1*tauf + 2*d1*tauf*tx_2 - 5*d1*dd*tauf*tz_2*sin(tz + tz_2*(d2*tauf^2 + d1*tauf)) - 10*d2*dd*tauf^2*tz_2*sin(tz + tz_2*(d2*tauf^2 + d1*tauf))))/(5*tauf^3))/(d1 + 2*d2*tau)^2 + (2*d2*(cx_2*d1 - (tau*(30*cx - 30*tx + 30*tauf^4*x4 + 30*tauf^5*x5 + 30*tauf^6*x6 + 30*tauf^7*x7 + 30*tauf^8*x8 + 30*tauf^9*x9 - 30*dd*cos(tz + tz_2*(d2*tauf^2 + d1*tauf)) + 11*d2*tauf^2*tx_2 + 20*cx_2*d1*tauf + d1*tauf*tx_2 - 10*d1*dd*tauf*tz_2*sin(tz + tz_2*(d2*tauf^2 + d1*tauf)) - 20*d2*dd*tauf^2*tz_2*sin(tz + tz_2*(d2*tauf^2 + d1*tauf))))/(5*tauf^2) + (3*tau^2*(10*cx - 10*tx + 10*tauf^4*x4 + 10*tauf^5*x5 + 10*tauf^6*x6 + 10*tauf^7*x7 + 10*tauf^8*x8 + 10*tauf^9*x9 - 10*dd*cos(tz + tz_2*(d2*tauf^2 + d1*tauf)) + 7*d2*tauf^2*tx_2 + 5*cx_2*d1*tauf + 2*d1*tauf*tx_2 - 5*d1*dd*tauf*tz_2*sin(tz + tz_2*(d2*tauf^2 + d1*tauf)) - 10*d2*dd*tauf^2*tz_2*sin(tz + tz_2*(d2*tauf^2 + d1*tauf))))/(5*tauf^3)))/(d1 + 2*d2*tau)^3);
            fy(i)= -m*(((30*cy - 30*ty - 30*dd*sin(tz + tz_2*(d2*tauf^2 + d1*tauf)) + 30*tauf^4*y4 + 30*tauf^5*y5 + 30*tauf^6*y6 + 30*tauf^7*y7 + 30*tauf^8*y8 + 30*tauf^9*y9 + 11*d2*tauf^2*ty_2 + 20*cy_2*d1*tauf + d1*tauf*ty_2 + 10*d1*dd*tauf*tz_2*sin(tz + tz_2*(d2*tauf^2 + d1*tauf)) + 20*d2*dd*tauf^2*tz_2*sin(tz + tz_2*(d2*tauf^2 + d1*tauf)))/(5*tauf^2) - (6*tau*(10*cy - 10*ty - 10*dd*sin(tz + tz_2*(d2*tauf^2 + d1*tauf)) + 10*tauf^4*y4 + 10*tauf^5*y5 + 10*tauf^6*y6 + 10*tauf^7*y7 + 10*tauf^8*y8 + 10*tauf^9*y9 + 7*d2*tauf^2*ty_2 + 5*cy_2*d1*tauf + 2*d1*tauf*ty_2 + 5*d1*dd*tauf*tz_2*sin(tz + tz_2*(d2*tauf^2 + d1*tauf)) + 10*d2*dd*tauf^2*tz_2*sin(tz + tz_2*(d2*tauf^2 + d1*tauf))))/(5*tauf^3))/(d1 + 2*d2*tau)^2 + (2*d2*(cy_2*d1 - (tau*(30*cy - 30*ty - 30*dd*sin(tz + tz_2*(d2*tauf^2 + d1*tauf)) + 30*tauf^4*y4 + 30*tauf^5*y5 + 30*tauf^6*y6 + 30*tauf^7*y7 + 30*tauf^8*y8 + 30*tauf^9*y9 + 11*d2*tauf^2*ty_2 + 20*cy_2*d1*tauf + d1*tauf*ty_2 + 10*d1*dd*tauf*tz_2*sin(tz + tz_2*(d2*tauf^2 + d1*tauf)) + 20*d2*dd*tauf^2*tz_2*sin(tz + tz_2*(d2*tauf^2 + d1*tauf))))/(5*tauf^2) + (3*tau^2*(10*cy - 10*ty - 10*dd*sin(tz + tz_2*(d2*tauf^2 + d1*tauf)) + 10*tauf^4*y4 + 10*tauf^5*y5 + 10*tauf^6*y6 + 10*tauf^7*y7 + 10*tauf^8*y8 + 10*tauf^9*y9 + 7*d2*tauf^2*ty_2 + 5*cy_2*d1*tauf + 2*d1*tauf*ty_2 + 5*d1*dd*tauf*tz_2*sin(tz + tz_2*(d2*tauf^2 + d1*tauf)) + 10*d2*dd*tauf^2*tz_2*sin(tz + tz_2*(d2*tauf^2 + d1*tauf))))/(5*tauf^3)))/(d1 + 2*d2*tau)^3);
            fz(i)= -Iz*(((2*(3*cz - 3*tz + 3*tauf^4*z4 + 3*tauf^5*z5 + 3*tauf^6*z6 + 3*tauf^7*z7 + 3*tauf^8*z8 + 3*tauf^9*z9 - d2*tauf^2*tz_2 + 2*cz_2*d1*tauf - 2*d1*tauf*tz_2))/tauf^2 - (6*tau*(2*cz - 2*tz + 2*tauf^4*z4 + 2*tauf^5*z5 + 2*tauf^6*z6 + 2*tauf^7*z7 + 2*tauf^8*z8 + 2*tauf^9*z9 + cz_2*d1*tauf - d1*tauf*tz_2))/tauf^3)/(d1 + 2*d2*tau)^2 + (2*d2*(cz_2*d1 - (2*tau*(3*cz - 3*tz + 3*tauf^4*z4 + 3*tauf^5*z5 + 3*tauf^6*z6 + 3*tauf^7*z7 + 3*tauf^8*z8 + 3*tauf^9*z9 - d2*tauf^2*tz_2 + 2*cz_2*d1*tauf - 2*d1*tauf*tz_2))/tauf^2 + (3*tau^2*(2*cz - 2*tz + 2*tauf^4*z4 + 2*tauf^5*z5 + 2*tauf^6*z6 + 2*tauf^7*z7 + 2*tauf^8*z8 + 2*tauf^9*z9 + cz_2*d1*tauf - d1*tauf*tz_2))/tauf^3))/(d1 + 2*d2*tau)^3);

            if s==1    % 1st run, calculate Ep with rp
                Ep(i)=(fx(i)^2+fy(i)^2+fz(i)^2);
            elseif s==2 % 2nd run, calculate En with rn
                En(i)=(fx(i)^2+fy(i)^2+fz(i)^2);
            end
        end 
    end
    gp=trapz(TAU,Ep.*(d1+2*d2*TAU));
    gn=trapz(TAU,En.*(d1+2*d2*TAU));
    dg(1,j)=(gp-gn)/(2*D(j));
end 

gg=dg';


end 
function h = findh(r, par) 

% Separating out the inputs (computational efficiency)
m=par(1);Iz=par(2);FXmax=par(3);FYmax=par(4);FZmax=par(5);dd=par(6); 
cx=par(7);cy=par(8);cz=par(9);cx_2=par(10);cy_2=par(11);cz_2=par(12);
tx=par(13);ty=par(14);tz=par(15);tx_2=par(16);ty_2=par(17);tz_2=par(18);
Tmax=par(19);fixed_att=par(20);

d1 = r(1); d2 = r(2); tauf = r(3); e_FX = r(4);
e_FY = r(5); e_TZ = r(6); u = r(7); e_t = r(8);
x4=r(9); x5=r(10); x6=r(11); x7=r(12); x8=r(13); x9=r(14);
y4=r(15); y5=r(16); y6=r(17); y7=r(18); y8=r(19); y9=r(20);
z4=r(21); z5=r(22); z6=r(23); z7=r(24); z8=r(25); z9=r(26);

%%
n=20;
TAU=[0:1/n:1]*tauf;
fx=zeros(1,length(TAU));fy=zeros(1,length(TAU));fz=zeros(1,length(TAU));
theta=zeros(1,length(TAU));h=zeros(5,1);
for i=1:length(TAU)
    tau=TAU(i);
    fx(i)= -m*(((30*cx - 30*tx + 30*tauf^4*x4 + 30*tauf^5*x5 + 30*tauf^6*x6 + 30*tauf^7*x7 + 30*tauf^8*x8 + 30*tauf^9*x9 - 30*dd*cos(tz + tz_2*(d2*tauf^2 + d1*tauf)) + 11*d2*tauf^2*tx_2 + 20*cx_2*d1*tauf + d1*tauf*tx_2 - 10*d1*dd*tauf*tz_2*sin(tz + tz_2*(d2*tauf^2 + d1*tauf)) - 20*d2*dd*tauf^2*tz_2*sin(tz + tz_2*(d2*tauf^2 + d1*tauf)))/(5*tauf^2) - (6*tau*(10*cx - 10*tx + 10*tauf^4*x4 + 10*tauf^5*x5 + 10*tauf^6*x6 + 10*tauf^7*x7 + 10*tauf^8*x8 + 10*tauf^9*x9 - 10*dd*cos(tz + tz_2*(d2*tauf^2 + d1*tauf)) + 7*d2*tauf^2*tx_2 + 5*cx_2*d1*tauf + 2*d1*tauf*tx_2 - 5*d1*dd*tauf*tz_2*sin(tz + tz_2*(d2*tauf^2 + d1*tauf)) - 10*d2*dd*tauf^2*tz_2*sin(tz + tz_2*(d2*tauf^2 + d1*tauf))))/(5*tauf^3))/(d1 + 2*d2*tau)^2 + (2*d2*(cx_2*d1 - (tau*(30*cx - 30*tx + 30*tauf^4*x4 + 30*tauf^5*x5 + 30*tauf^6*x6 + 30*tauf^7*x7 + 30*tauf^8*x8 + 30*tauf^9*x9 - 30*dd*cos(tz + tz_2*(d2*tauf^2 + d1*tauf)) + 11*d2*tauf^2*tx_2 + 20*cx_2*d1*tauf + d1*tauf*tx_2 - 10*d1*dd*tauf*tz_2*sin(tz + tz_2*(d2*tauf^2 + d1*tauf)) - 20*d2*dd*tauf^2*tz_2*sin(tz + tz_2*(d2*tauf^2 + d1*tauf))))/(5*tauf^2) + (3*tau^2*(10*cx - 10*tx + 10*tauf^4*x4 + 10*tauf^5*x5 + 10*tauf^6*x6 + 10*tauf^7*x7 + 10*tauf^8*x8 + 10*tauf^9*x9 - 10*dd*cos(tz + tz_2*(d2*tauf^2 + d1*tauf)) + 7*d2*tauf^2*tx_2 + 5*cx_2*d1*tauf + 2*d1*tauf*tx_2 - 5*d1*dd*tauf*tz_2*sin(tz + tz_2*(d2*tauf^2 + d1*tauf)) - 10*d2*dd*tauf^2*tz_2*sin(tz + tz_2*(d2*tauf^2 + d1*tauf))))/(5*tauf^3)))/(d1 + 2*d2*tau)^3);
    fy(i)= -m*(((30*cy - 30*ty - 30*dd*sin(tz + tz_2*(d2*tauf^2 + d1*tauf)) + 30*tauf^4*y4 + 30*tauf^5*y5 + 30*tauf^6*y6 + 30*tauf^7*y7 + 30*tauf^8*y8 + 30*tauf^9*y9 + 11*d2*tauf^2*ty_2 + 20*cy_2*d1*tauf + d1*tauf*ty_2 + 10*d1*dd*tauf*tz_2*sin(tz + tz_2*(d2*tauf^2 + d1*tauf)) + 20*d2*dd*tauf^2*tz_2*sin(tz + tz_2*(d2*tauf^2 + d1*tauf)))/(5*tauf^2) - (6*tau*(10*cy - 10*ty - 10*dd*sin(tz + tz_2*(d2*tauf^2 + d1*tauf)) + 10*tauf^4*y4 + 10*tauf^5*y5 + 10*tauf^6*y6 + 10*tauf^7*y7 + 10*tauf^8*y8 + 10*tauf^9*y9 + 7*d2*tauf^2*ty_2 + 5*cy_2*d1*tauf + 2*d1*tauf*ty_2 + 5*d1*dd*tauf*tz_2*sin(tz + tz_2*(d2*tauf^2 + d1*tauf)) + 10*d2*dd*tauf^2*tz_2*sin(tz + tz_2*(d2*tauf^2 + d1*tauf))))/(5*tauf^3))/(d1 + 2*d2*tau)^2 + (2*d2*(cy_2*d1 - (tau*(30*cy - 30*ty - 30*dd*sin(tz + tz_2*(d2*tauf^2 + d1*tauf)) + 30*tauf^4*y4 + 30*tauf^5*y5 + 30*tauf^6*y6 + 30*tauf^7*y7 + 30*tauf^8*y8 + 30*tauf^9*y9 + 11*d2*tauf^2*ty_2 + 20*cy_2*d1*tauf + d1*tauf*ty_2 + 10*d1*dd*tauf*tz_2*sin(tz + tz_2*(d2*tauf^2 + d1*tauf)) + 20*d2*dd*tauf^2*tz_2*sin(tz + tz_2*(d2*tauf^2 + d1*tauf))))/(5*tauf^2) + (3*tau^2*(10*cy - 10*ty - 10*dd*sin(tz + tz_2*(d2*tauf^2 + d1*tauf)) + 10*tauf^4*y4 + 10*tauf^5*y5 + 10*tauf^6*y6 + 10*tauf^7*y7 + 10*tauf^8*y8 + 10*tauf^9*y9 + 7*d2*tauf^2*ty_2 + 5*cy_2*d1*tauf + 2*d1*tauf*ty_2 + 5*d1*dd*tauf*tz_2*sin(tz + tz_2*(d2*tauf^2 + d1*tauf)) + 10*d2*dd*tauf^2*tz_2*sin(tz + tz_2*(d2*tauf^2 + d1*tauf))))/(5*tauf^3)))/(d1 + 2*d2*tau)^3);
    fz(i)= -Iz*(((2*(3*cz - 3*tz + 3*tauf^4*z4 + 3*tauf^5*z5 + 3*tauf^6*z6 + 3*tauf^7*z7 + 3*tauf^8*z8 + 3*tauf^9*z9 - d2*tauf^2*tz_2 + 2*cz_2*d1*tauf - 2*d1*tauf*tz_2))/tauf^2 - (6*tau*(2*cz - 2*tz + 2*tauf^4*z4 + 2*tauf^5*z5 + 2*tauf^6*z6 + 2*tauf^7*z7 + 2*tauf^8*z8 + 2*tauf^9*z9 + cz_2*d1*tauf - d1*tauf*tz_2))/tauf^3)/(d1 + 2*d2*tau)^2 + (2*d2*(cz_2*d1 - (2*tau*(3*cz - 3*tz + 3*tauf^4*z4 + 3*tauf^5*z5 + 3*tauf^6*z6 + 3*tauf^7*z7 + 3*tauf^8*z8 + 3*tauf^9*z9 - d2*tauf^2*tz_2 + 2*cz_2*d1*tauf - 2*d1*tauf*tz_2))/tauf^2 + (3*tau^2*(2*cz - 2*tz + 2*tauf^4*z4 + 2*tauf^5*z5 + 2*tauf^6*z6 + 2*tauf^7*z7 + 2*tauf^8*z8 + 2*tauf^9*z9 + cz_2*d1*tauf - d1*tauf*tz_2))/tauf^3))/(d1 + 2*d2*tau)^3);
    theta(i)= cz + ((d2*tau^2 + d1*tau)^3*(2*cz - 2*tz + 2*tauf^4*z4 + 2*tauf^5*z5 + 2*tauf^6*z6 + 2*tauf^7*z7 + 2*tauf^8*z8 + 2*tauf^9*z9 + cz_2*d1*tauf - d1*tauf*tz_2))/tauf^3 - ((d2*tau^2 + d1*tau)^2*(3*cz - 3*tz + 3*tauf^4*z4 + 3*tauf^5*z5 + 3*tauf^6*z6 + 3*tauf^7*z7 + 3*tauf^8*z8 + 3*tauf^9*z9 - d2*tauf^2*tz_2 + 2*cz_2*d1*tauf - 2*d1*tauf*tz_2))/tauf^2 + cz_2*d1*(d2*tau^2 + d1*tau);
end
h(1,1)=e_FX^2-FXmax^2+max((fx.*cos(theta)+fy.*sin(theta)).^2);

h(2,1)=e_FY^2-FYmax^2+max((-fx.*sin(theta)+fy.*cos(theta)).^2);

h(3,1)=e_TZ^2-FZmax^2+max(fz.^2);

h(4,1)=tauf-u^2;

h(5,1)=d1*tauf+d2*tauf^2+e_t^2-Tmax;

%h=h;

end
function hg = findhg(r,par)

% Separating out the inputs (computational efficiency)
m=par(1);Iz=par(2);FXmax=par(3);FYmax=par(4);FZmax=par(5);dd=par(6); 
cx=par(7);cy=par(8);cz=par(9);cx_2=par(10);cy_2=par(11);cz_2=par(12);
tx=par(13);ty=par(14);tz=par(15);tx_2=par(16);ty_2=par(17);tz_2=par(18);
Tmax=par(19);fixed_att=par(20);

%%
r = r';
r0 = r;
D=abs(r/1000)+0.0001;
dh=zeros(5,length(D));
for j=1:length(r)
    rp=r0; rn=r0;
    rp(j)=rp(j)+D(j);rn(j)=rn(j)-D(j);
    rpn=[rp;rn]; 
    hp=zeros(5,1);hn=zeros(5,1); 
    for k=1:2
        r=rpn(k,:);
        d1 = r(1); d2 = r(2); tauf = r(3); e_FX = r(4);
        e_FY = r(5); e_TZ = r(6); u = r(7); e_t = r(8);
        x4=r(9); x5=r(10); x6=r(11); x7=r(12); x8=r(13); x9=r(14);
        y4=r(15); y5=r(16); y6=r(17); y7=r(18); y8=r(19); y9=r(20);
        z4=r(21); z5=r(22); z6=r(23); z7=r(24); z8=r(25); z9=r(26);
        
        n=20;
        TAU=(0:1/n:1)*tauf;
        fx=zeros(1,length(TAU));fy=zeros(1,length(TAU));fz=zeros(1,length(TAU));
        theta=zeros(1,length(TAU));
        for i=1:length(TAU)
            tau=TAU(i);
            fx(i)= -m*(((30*cx - 30*tx + 30*tauf^4*x4 + 30*tauf^5*x5 + 30*tauf^6*x6 + 30*tauf^7*x7 + 30*tauf^8*x8 + 30*tauf^9*x9 - 30*dd*cos(tz + tz_2*(d2*tauf^2 + d1*tauf)) + 11*d2*tauf^2*tx_2 + 20*cx_2*d1*tauf + d1*tauf*tx_2 - 10*d1*dd*tauf*tz_2*sin(tz + tz_2*(d2*tauf^2 + d1*tauf)) - 20*d2*dd*tauf^2*tz_2*sin(tz + tz_2*(d2*tauf^2 + d1*tauf)))/(5*tauf^2) - (6*tau*(10*cx - 10*tx + 10*tauf^4*x4 + 10*tauf^5*x5 + 10*tauf^6*x6 + 10*tauf^7*x7 + 10*tauf^8*x8 + 10*tauf^9*x9 - 10*dd*cos(tz + tz_2*(d2*tauf^2 + d1*tauf)) + 7*d2*tauf^2*tx_2 + 5*cx_2*d1*tauf + 2*d1*tauf*tx_2 - 5*d1*dd*tauf*tz_2*sin(tz + tz_2*(d2*tauf^2 + d1*tauf)) - 10*d2*dd*tauf^2*tz_2*sin(tz + tz_2*(d2*tauf^2 + d1*tauf))))/(5*tauf^3))/(d1 + 2*d2*tau)^2 + (2*d2*(cx_2*d1 - (tau*(30*cx - 30*tx + 30*tauf^4*x4 + 30*tauf^5*x5 + 30*tauf^6*x6 + 30*tauf^7*x7 + 30*tauf^8*x8 + 30*tauf^9*x9 - 30*dd*cos(tz + tz_2*(d2*tauf^2 + d1*tauf)) + 11*d2*tauf^2*tx_2 + 20*cx_2*d1*tauf + d1*tauf*tx_2 - 10*d1*dd*tauf*tz_2*sin(tz + tz_2*(d2*tauf^2 + d1*tauf)) - 20*d2*dd*tauf^2*tz_2*sin(tz + tz_2*(d2*tauf^2 + d1*tauf))))/(5*tauf^2) + (3*tau^2*(10*cx - 10*tx + 10*tauf^4*x4 + 10*tauf^5*x5 + 10*tauf^6*x6 + 10*tauf^7*x7 + 10*tauf^8*x8 + 10*tauf^9*x9 - 10*dd*cos(tz + tz_2*(d2*tauf^2 + d1*tauf)) + 7*d2*tauf^2*tx_2 + 5*cx_2*d1*tauf + 2*d1*tauf*tx_2 - 5*d1*dd*tauf*tz_2*sin(tz + tz_2*(d2*tauf^2 + d1*tauf)) - 10*d2*dd*tauf^2*tz_2*sin(tz + tz_2*(d2*tauf^2 + d1*tauf))))/(5*tauf^3)))/(d1 + 2*d2*tau)^3);
            fy(i)= -m*(((30*cy - 30*ty - 30*dd*sin(tz + tz_2*(d2*tauf^2 + d1*tauf)) + 30*tauf^4*y4 + 30*tauf^5*y5 + 30*tauf^6*y6 + 30*tauf^7*y7 + 30*tauf^8*y8 + 30*tauf^9*y9 + 11*d2*tauf^2*ty_2 + 20*cy_2*d1*tauf + d1*tauf*ty_2 + 10*d1*dd*tauf*tz_2*sin(tz + tz_2*(d2*tauf^2 + d1*tauf)) + 20*d2*dd*tauf^2*tz_2*sin(tz + tz_2*(d2*tauf^2 + d1*tauf)))/(5*tauf^2) - (6*tau*(10*cy - 10*ty - 10*dd*sin(tz + tz_2*(d2*tauf^2 + d1*tauf)) + 10*tauf^4*y4 + 10*tauf^5*y5 + 10*tauf^6*y6 + 10*tauf^7*y7 + 10*tauf^8*y8 + 10*tauf^9*y9 + 7*d2*tauf^2*ty_2 + 5*cy_2*d1*tauf + 2*d1*tauf*ty_2 + 5*d1*dd*tauf*tz_2*sin(tz + tz_2*(d2*tauf^2 + d1*tauf)) + 10*d2*dd*tauf^2*tz_2*sin(tz + tz_2*(d2*tauf^2 + d1*tauf))))/(5*tauf^3))/(d1 + 2*d2*tau)^2 + (2*d2*(cy_2*d1 - (tau*(30*cy - 30*ty - 30*dd*sin(tz + tz_2*(d2*tauf^2 + d1*tauf)) + 30*tauf^4*y4 + 30*tauf^5*y5 + 30*tauf^6*y6 + 30*tauf^7*y7 + 30*tauf^8*y8 + 30*tauf^9*y9 + 11*d2*tauf^2*ty_2 + 20*cy_2*d1*tauf + d1*tauf*ty_2 + 10*d1*dd*tauf*tz_2*sin(tz + tz_2*(d2*tauf^2 + d1*tauf)) + 20*d2*dd*tauf^2*tz_2*sin(tz + tz_2*(d2*tauf^2 + d1*tauf))))/(5*tauf^2) + (3*tau^2*(10*cy - 10*ty - 10*dd*sin(tz + tz_2*(d2*tauf^2 + d1*tauf)) + 10*tauf^4*y4 + 10*tauf^5*y5 + 10*tauf^6*y6 + 10*tauf^7*y7 + 10*tauf^8*y8 + 10*tauf^9*y9 + 7*d2*tauf^2*ty_2 + 5*cy_2*d1*tauf + 2*d1*tauf*ty_2 + 5*d1*dd*tauf*tz_2*sin(tz + tz_2*(d2*tauf^2 + d1*tauf)) + 10*d2*dd*tauf^2*tz_2*sin(tz + tz_2*(d2*tauf^2 + d1*tauf))))/(5*tauf^3)))/(d1 + 2*d2*tau)^3);
            fz(i)= -Iz*(((2*(3*cz - 3*tz + 3*tauf^4*z4 + 3*tauf^5*z5 + 3*tauf^6*z6 + 3*tauf^7*z7 + 3*tauf^8*z8 + 3*tauf^9*z9 - d2*tauf^2*tz_2 + 2*cz_2*d1*tauf - 2*d1*tauf*tz_2))/tauf^2 - (6*tau*(2*cz - 2*tz + 2*tauf^4*z4 + 2*tauf^5*z5 + 2*tauf^6*z6 + 2*tauf^7*z7 + 2*tauf^8*z8 + 2*tauf^9*z9 + cz_2*d1*tauf - d1*tauf*tz_2))/tauf^3)/(d1 + 2*d2*tau)^2 + (2*d2*(cz_2*d1 - (2*tau*(3*cz - 3*tz + 3*tauf^4*z4 + 3*tauf^5*z5 + 3*tauf^6*z6 + 3*tauf^7*z7 + 3*tauf^8*z8 + 3*tauf^9*z9 - d2*tauf^2*tz_2 + 2*cz_2*d1*tauf - 2*d1*tauf*tz_2))/tauf^2 + (3*tau^2*(2*cz - 2*tz + 2*tauf^4*z4 + 2*tauf^5*z5 + 2*tauf^6*z6 + 2*tauf^7*z7 + 2*tauf^8*z8 + 2*tauf^9*z9 + cz_2*d1*tauf - d1*tauf*tz_2))/tauf^3))/(d1 + 2*d2*tau)^3);
            theta(i)= cz + ((d2*tau^2 + d1*tau)^3*(2*cz - 2*tz + 2*tauf^4*z4 + 2*tauf^5*z5 + 2*tauf^6*z6 + 2*tauf^7*z7 + 2*tauf^8*z8 + 2*tauf^9*z9 + cz_2*d1*tauf - d1*tauf*tz_2))/tauf^3 - ((d2*tau^2 + d1*tau)^2*(3*cz - 3*tz + 3*tauf^4*z4 + 3*tauf^5*z5 + 3*tauf^6*z6 + 3*tauf^7*z7 + 3*tauf^8*z8 + 3*tauf^9*z9 - d2*tauf^2*tz_2 + 2*cz_2*d1*tauf - 2*d1*tauf*tz_2))/tauf^2 + cz_2*d1*(d2*tau^2 + d1*tau);

        end
        if k==1
            hp(1,1)=e_FX^2-FXmax^2+max((fx.*cos(theta)+fy.*sin(theta)).^2);

            hp(2,1)=e_FY^2-FYmax^2+max((-fx.*sin(theta)+fy.*cos(theta)).^2);

            hp(3,1)=e_TZ^2-FZmax^2+max(fz.^2);

            hp(4,1)=tauf-u^2;

            hp(5,1)=d1*tauf+d2*tauf^2+e_t^2-Tmax;
        elseif k==2
            hn(1,1)=e_FX^2-FXmax^2+max((fx.*cos(theta)+fy.*sin(theta)).^2);

            hn(2,1)=e_FY^2-FYmax^2+max((-fx.*sin(theta)+fy.*cos(theta)).^2);

            hn(3,1)=e_TZ^2-FZmax^2+max(fz.^2);

            hn(4,1)=tauf-u^2;

            hn(5,1)=d1*tauf+d2*tauf^2+e_t^2-Tmax;
        end
    end
    for i=1:length(hn)
        dh(i,j)=(hp(i)-hn(i))/(2*D(j));
    end
end
hg=dh';

end  
%%%%%%%%%%%%%%%%%%%%%%%%%%%%%%%%%%%%%%%%%%%%%%%%%%%%%%%%%%%%%%%%%%%%%%%%%%%

== matlab function IDVDSGRA_StatObs_Close/Phase #3: Experiment/Change RED Behavior/Sub-Phase #3 /Hough Control/MATLAB Function2 ==
  data: Oy output; z input; Ox output
function [Oy, Ox]   = C3( z )
%C3 gives the rotation matrix about the z-axis for an angle 'z'
%   z - the angle about the z-axis which you rotate
%   A - the rotation matrix

Ox = [cos(z) sin(z); -sin(z) cos(z)]*[1;0];
Oy = [cos(z) sin(z); -sin(z) cos(z)]*[0;1];
end

== matlab function IDVDSGRA_StatObs_Close/Phase #3: Experiment/Change RED Behavior/Sub-Phase #3 /Hough Control/MATLAB Function3 ==
  data: z input; Ox output
function Ox    = C3( z )
%C3 gives the rotation matrix about the z-axis for an angle 'z'
%   z - the angle about the z-axis which you rotate
%   A - the rotation matrix

Ox = [cos(z) sin(z); -sin(z) cos(z)]*[1;0];
end

== matlab function IDVDSGRA_StatObs_Close/Phase #3: Experiment/Change RED Behavior/Sub-Phase #3 /Hough Control/MATLAB Function4 ==
  data: Oy input; e_out output; e_in input
function e_out = fcn(Oy, e_in)

a = sign(Oy'*e_in);
e_out = -a*norm(e_in);

== matlab function IDVDSGRA_StatObs_Close/Phase #3: Experiment/Change BLACK Behavior/Sub-Phase #3 /Hough Control/MATLAB Function2 ==
  data: Oy output; z input; Ox output
function [Oy, Ox]   = C3( z )
%C3 gives the rotation matrix about the z-axis for an angle 'z'
%   z - the angle about the z-axis which you rotate
%   A - the rotation matrix

Ox = [cos(z) sin(z); -sin(z) cos(z)]*[1;0];
Oy = [cos(z) sin(z); -sin(z) cos(z)]*[0;1];
end

== matlab function IDVDSGRA_StatObs_Close/Phase #3: Experiment/Change BLACK Behavior/Sub-Phase #3 /Hough Control/MATLAB Function3 ==
  data: z input; Ox output
function Ox    = C3( z )
%C3 gives the rotation matrix about the z-axis for an angle 'z'
%   z - the angle about the z-axis which you rotate
%   A - the rotation matrix

Ox = [cos(z) sin(z); -sin(z) cos(z)]*[1;0];
end

== matlab function IDVDSGRA_StatObs_Close/Phase #3: Experiment/Change RED Behavior/Sub-Phase #1/Hough Control/MATLAB Function2 ==
  data: Oy output; z input; Ox output
function [Oy, Ox]   = C3( z )
%C3 gives the rotation matrix about the z-axis for an angle 'z'
%   z - the angle about the z-axis which you rotate
%   A - the rotation matrix

Ox = [cos(z) sin(z); -sin(z) cos(z)]*[1;0];
Oy = [cos(z) sin(z); -sin(z) cos(z)]*[0;1];
end

== matlab function IDVDSGRA_StatObs_Close/Phase #3: Experiment/Change RED Behavior/Sub-Phase #1/Hough Control/MATLAB Function3 ==
  data: z input; Ox output
function Ox    = C3( z )
%C3 gives the rotation matrix about the z-axis for an angle 'z'
%   z - the angle about the z-axis which you rotate
%   A - the rotation matrix

Ox = [cos(z) sin(z); -sin(z) cos(z)]*[1;0];
end

== matlab function IDVDSGRA_StatObs_Close/Phase #3: Experiment/Change RED Behavior/Sub-Phase #1/Hough Control/MATLAB Function4 ==
  data: Oy input; e_out output; e_in input
function e_out = fcn(Oy, e_in)

a = sign(Oy'*e_in);
e_out = -a*norm(e_in);

== matlab function IDVDSGRA_StatObs_Close/Phase #3: Experiment/Change BLACK Behavior/Sub-Phase #3 /Hough Control/MATLAB Function4 ==
  data: Oy input; e_out output; e_in input
function e_out = fcn(Oy, e_in)

a = sign(Oy'*e_in);
e_out = -a*norm(e_in);

== matlab function IDVDSGRA_StatObs_Close/Phase #3: Experiment/Change BLACK Behavior/Sub-Phase #2 /Hough Control/MATLAB Function2 ==
  data: Oy output; z input; Ox output
function [Oy, Ox]   = C3( z )
%C3 gives the rotation matrix about the z-axis for an angle 'z'
%   z - the angle about the z-axis which you rotate
%   A - the rotation matrix

Ox = [cos(z) sin(z); -sin(z) cos(z)]*[1;0];
Oy = [cos(z) sin(z); -sin(z) cos(z)]*[0;1];
end

== matlab function IDVDSGRA_StatObs_Close/Phase #3: Experiment/Change BLACK Behavior/Sub-Phase #2 /Hough Control/MATLAB Function3 ==
  data: z input; Ox output
function Ox    = C3( z )
%C3 gives the rotation matrix about the z-axis for an angle 'z'
%   z - the angle about the z-axis which you rotate
%   A - the rotation matrix

Ox = [cos(z) sin(z); -sin(z) cos(z)]*[1;0];
end

== matlab function IDVDSGRA_StatObs_Close/Phase #3: Experiment/Change RED Behavior/Sub-Phase #4/Hough Control/MATLAB Function2 ==
  data: Oy output; z input; Ox output
function [Oy, Ox]   = C3( z )
%C3 gives the rotation matrix about the z-axis for an angle 'z'
%   z - the angle about the z-axis which you rotate
%   A - the rotation matrix

Ox = [cos(z) sin(z); -sin(z) cos(z)]*[1;0];
Oy = [cos(z) sin(z); -sin(z) cos(z)]*[0;1];
end

== matlab function IDVDSGRA_StatObs_Close/Phase #3: Experiment/Change RED Behavior/Sub-Phase #4/Hough Control/MATLAB Function3 ==
  data: z input; Ox output
function Ox    = C3( z )
%C3 gives the rotation matrix about the z-axis for an angle 'z'
%   z - the angle about the z-axis which you rotate
%   A - the rotation matrix

Ox = [cos(z) sin(z); -sin(z) cos(z)]*[1;0];
end

== matlab function IDVDSGRA_StatObs_Close/Phase #3: Experiment/Change RED Behavior/Sub-Phase #4/Hough Control/MATLAB Function4 ==
  data: Oy input; e_out output; e_in input
function e_out = fcn(Oy, e_in)

a = sign(Oy'*e_in);
e_out = -a*norm(e_in);

== matlab function IDVDSGRA_StatObs_Close/Phase #3: Experiment/Change BLACK Behavior/Sub-Phase #4/Hough Control/MATLAB Function4 ==
  data: Oy input; e_out output; e_in input
function e_out = fcn(Oy, e_in)

a = sign(Oy'*e_in);
e_out = -a*norm(e_in);

== matlab function IDVDSGRA_StatObs_Close/Phase #3: Experiment/Change BLACK Behavior/Sub-Phase #1/Hough Control/MATLAB Function2 ==
  data: Oy output; z input; Ox output
function [Oy, Ox]   = C3( z )
%C3 gives the rotation matrix about the z-axis for an angle 'z'
%   z - the angle about the z-axis which you rotate
%   A - the rotation matrix

Ox = [cos(z) sin(z); -sin(z) cos(z)]*[1;0];
Oy = [cos(z) sin(z); -sin(z) cos(z)]*[0;1];
end

== matlab function IDVDSGRA_StatObs_Close/Phase #3: Experiment/Change BLACK Behavior/Sub-Phase #1/Hough Control/MATLAB Function3 ==
  data: z input; Ox output
function Ox    = C3( z )
%C3 gives the rotation matrix about the z-axis for an angle 'z'
%   z - the angle about the z-axis which you rotate
%   A - the rotation matrix

Ox = [cos(z) sin(z); -sin(z) cos(z)]*[1;0];
end

== matlab function IDVDSGRA_StatObs_Close/Phase #3: Experiment/Change BLACK Behavior/Sub-Phase #1/Hough Control/MATLAB Function4 ==
  data: Oy input; e_out output; e_in input
function e_out = fcn(Oy, e_in)

a = sign(Oy'*e_in);
e_out = -a*norm(e_in);

== matlab function IDVDSGRA_StatObs_Close/Phase #3: Experiment/Change BLACK Behavior/Sub-Phase #2 /Hough Control/MATLAB Function4 ==
  data: Oy input; e_out output; e_in input
function e_out = fcn(Oy, e_in)

a = sign(Oy'*e_in);
e_out = -a*norm(e_in);

== matlab function IDVDSGRA_StatObs_Close/Phase #5: Hold Home/Change BLACK Behavior/Hough Control/MATLAB Function2 ==
  data: Oy output; z input; Ox output
function [Oy, Ox]   = C3( z )
%C3 gives the rotation matrix about the z-axis for an angle 'z'
%   z - the angle about the z-axis which you rotate
%   A - the rotation matrix

Ox = [cos(z) sin(z); -sin(z) cos(z)]*[1;0];
Oy = [cos(z) sin(z); -sin(z) cos(z)]*[0;1];
end
